simulink model "BF_Q3"  (R2025b)
settings: Solver=VariableStepAuto  StartTime=0.0  StopTime=2000  RelTol=1e-3
values from neighbouring files (symbols this model uses):
  m_value = 50    [Dev_04_M.m]
undefined symbols (not defined in the file or in its folder): den_m, den_u, num_m, num_u
settings Model: Creator=Louis  LastModifiedBy=diegoalfonsocosta

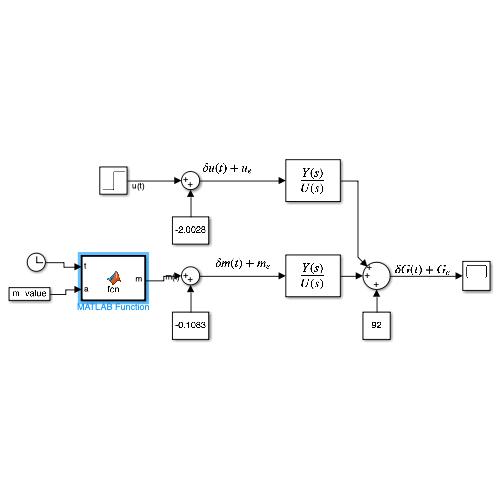
[thumbnail: Simulink's stored preview of the top-level diagram]
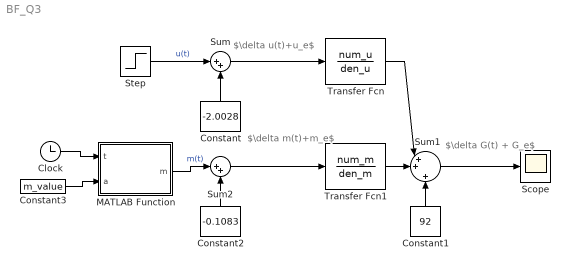
== system BF_Q3 ==
  note: $\delta G(t) + G_e$
  note: $\delta u(t)+u_e$
  note: $\delta m(t)+m_e$
  Clock : Clock
  Constant : Constant  Value=-2.0028
  Constant1 : Constant  Value=92
  Constant2 : Constant  Value=-0.1083
  Constant3 : Constant  Value=m_value
  MATLAB Function : MATLAB Function  TreatAsAtomicUnit=on
  Scope : Scope
      settings: ActiveDisplayYMinimum=-1  ActiveDisplayYMaximum=1  DataLoggingVariableName=GBF_Q3  DataLoggingSaveFormat=Array
  Step : Step  Time=0  After=2  SampleTime=0
  Sum : Sum  Inputs=|++
  Sum1 : Sum  Inputs=|++|+
  Sum2 : Sum  Inputs=|++
  Transfer Fcn : TransferFcn  Numerator=num_u  Denominator=den_u
  Transfer Fcn1 : TransferFcn  Numerator=num_m  Denominator=den_m
  wires:
  Step/1 -> Sum/1  "u(t)"
  Sum/1 -> Transfer Fcn/1
  Constant/1 -> Sum/2
  Transfer Fcn/1 -> Sum1/1
  Constant1/1 -> Sum1/3
  Sum1/1 -> Scope/1
  Constant2/1 -> Sum2/2
  Sum2/1 -> Transfer Fcn1/1
  Transfer Fcn1/1 -> Sum1/2
  Clock/1 -> MATLAB Function/1(t)
  MATLAB Function/1(m) -> Sum2/1  "m(t)"
  Constant3/1 -> MATLAB Function/2(a)

== matlab function BF_Q3/MATLAB Function ==
  data: t input; m output; a input
function m = fcn(t,a)

if (t >= 0 && t <= a)
    m = a;

else
    m = 0;
end
